simulink model "lookup_table_2D"  (R2021a)
settings: Solver=VariableStepAuto  StartTime=0.0  StopTime=10.0  RelTol=1e-3
libraries: simulink x1
settings Model: Creator=Acer  LastModifiedBy=Acer

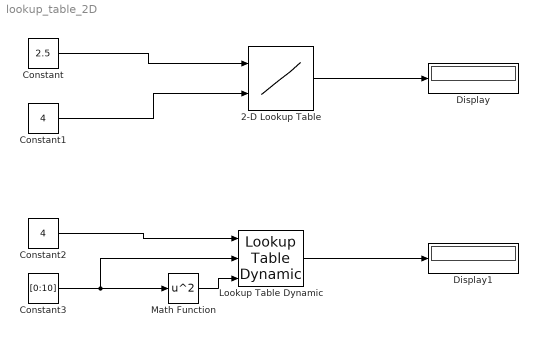
== system lookup_table_2D ==
  2-D Lookup Table : Lookup_n-D  BreakpointsForDimension1=[1:3]  BreakpointsForDimension2=[1:4]  Table=[2 3 4 5;3 4 5 6;4 5 6 7]  InternalRulePriority=Speed  RndMeth=Simplest  InputSameDT=on
      settings: InputPortMap=u0,u1
  Constant : Constant  Value=2.5
  Constant1 : Constant  Value=4
  Constant2 : Constant  Value=4
  Constant3 : Constant  Value=[0:10]
  Display : Display
  Display1 : Display
  Lookup Table Dynamic : simulink/Lookup Tables/Lookup Table Dynamic  LookUpMeth=Interpolation-Use End Values  OutDataType=fixdt('double')  OutScaling=2^-10  OutputDataTypeScalingMode=Specify via dialog  OutDataTypeStr=double  DoSatur=off
  Math Function : Math  Operator=square  SaturateOnIntegerOverflow=on
  wires:
  Constant/1 -> 2-D Lookup Table/1
  Constant1/1 -> 2-D Lookup Table/2
  2-D Lookup Table/1 -> Display/1
  Constant2/1 -> Lookup Table Dynamic/1
  Constant3/1 -> Math Function/1, Lookup Table Dynamic/2
  Math Function/1 -> Lookup Table Dynamic/3
  Lookup Table Dynamic/1 -> Display1/1
